simulink model "System"  (R2024a)
settings: Solver=VariableStepAuto  StartTime=0.0  StopTime=10.0  RelTol=1e-3
libraries: neural x2
settings Model: Creator=max11mus  LastModifiedBy=max11mus

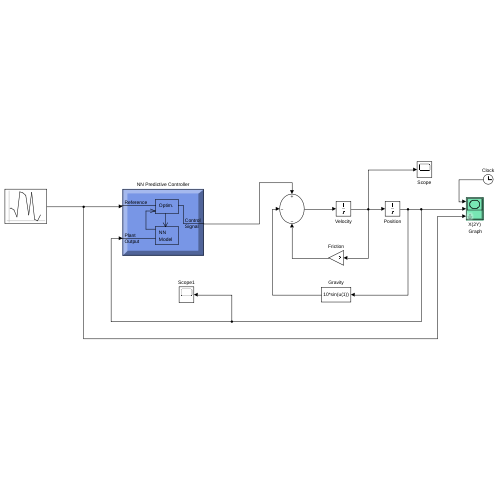
[thumbnail: Simulink's stored preview of the top-level diagram]
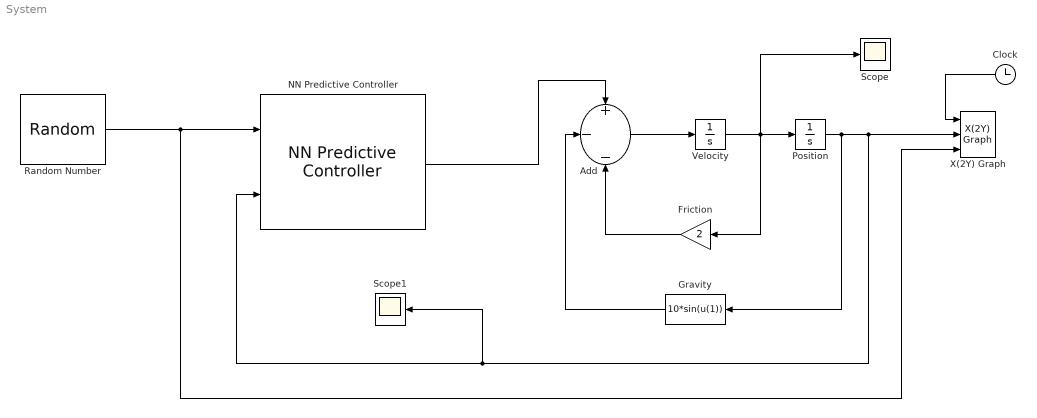
== system System ==
  Add : Sum  Inputs=+||-||-
  Clock : Clock
  Friction : Gain  Gain=2
  Gravity : Fcn  Expr=10*sin(u(1))
  NN Predictive Controller : neural/Control Systems/NN Predictive Controller  epochs=10  minp=-14.860973275977976016  maxp=14.972411842840820384  mint=-3.2887980026526069111  maxt=14.972411842840820384  Normalize=0  IW=[-0.032209844966698181201 0.0004842303811762906085 -0.038214774508017898547 0.087891959742595143767 -0.0049186837795332106343;-0.0037266038644475137781 -0.0053214205196589073679 0.006700009668674138455 0.0050755072350715437629 -0.0090455928933601964514;-0.0072756233672057243206 0.020376661347633842625 -0.033005692527208564668 0.010347523880553283898 0.036857966345246385986;-0.00038199302969159549571 -0.0059612728941718946124 0.013388867166121689797 -0.010360796205912608386 0.003487135037739601956;-0.0046614812815905194363 -0.0028269766095801204635 0.00030057352605401246783 0.0064554017982060268172 -0.0022030445024334051329;-0.0094467253000392586298 -0.0042207140094451646786 0.045248285726168152587 -0.025888487260812172164 -0.002820999804125486933;0.065543385541593959798 -0.0016025414154424494004 -0.0084955300195080837855 0.044609410010118671908 -0.26853262779806130744;0.017946126289430236467 -0.015971807856565621575 -0.0070211617130560765795 0.011444625729904966266 0.010874294340424636024;-0.0021688861781463536493 -0.0035622984387113317863 0.040072202786979448097 -0.018852965401898433978 -0.012267489590222301066;-0.0025428786120997304288 -0.0071555839750277652062 0.0052904364999521507826 0.004310034030136751515 -0.0029703349926871033468;0.007186386802497442966 0.0041023569100574761373 0.00068661195843568991956 -0.016977898377474390235 0.011745413647987718725;0.1130291466453810928 0.1847423194375882316 0.023123739836479410836 -0.2623344344032326747 -0.018356815139350751709;0.027774236790948012704 0.0028672682886705753644 0.015458774845652670932 -0.062765193394395860094 0.0054360877460552028961;0.0067224951938523978823 0.00083501283958491764187 -0.001283833296912832711 -0.012041984208070262777 0.0029837734768752635639;0.0069680791525584253807 -0.0044436167500601416597 0.0051584966512181230913 -0.014238832458994900992 -0.0051929494639878339204]  LW1_2=[-0.26243930864913889156 -0.12520756836498139752 -0.049859422322473881395 -0.0032752693913916230278 -0.21877664073705208048;-0.085553520951359610103 0.27651015843062082267 0.33749027304918660652 0.11372350823367174955 -0.13998821343616371649;-0.051262059060211306871 0.14553524371126419501 0.012158167251771118816 0.13234730689237414469 -0.31692057220921582283;-0.1659611043529373442 -0.22867683011507383695 -0.12064160820941764729 -0.25555605197606945378 0.47379167540947147996;-0.16667829573614167948 -0.14623179297968696977 -0.17550654818669228496 0.086019591308161766352 0.17447895641370442243;0.13273667574946193537 0.27597615594842184183 -0.12052646882881125345 0.15989614547386321597 -0.190668955400320278;0.013209872517279412987 0.17507718552719539473 -0.24607151945859806474 -0.084451465827836177946 -0.038421568456381463563;0.056189912372349971881 -0.19741810753112501442 0.015606879920724505903 0.023964644441251702067 0.24055696827493480705;0.25649967909796261845 0.053178233680966843777 0.18535281867337646822 -0.15204179248997790053 -0.10986325716373966654;-0.33505348193771761212 -0.19627538603327043809 0.130437673814499 -0.0097946347635215723348 0.12477419649646211142;0.14084781289795461623 -0.28347782651436276291 -0.28700933543676010462 0.1780649036607043767 -0.085136284393081823607;-0.2000008205941552486 -0.140154005050131647 0.027358468624533813923 0.072417932615793628726 -0.18151652074197416331;-0.26712085242982885891 0.17012835486666119666 0.16455985338081091651 0.20377306294523389596 -0.031959636277844219454;-0.28621748767442251049 -0.33565539170103531053 0.10951369435619884296 -0.28397325867506717501 0.36987661197218385523;-0.34568323062985784055 0.19495674497156445515 -0.33771385385234831134 -0.17879254297502281124 0.18187340190716883015]  LW2_1=[-0.19670780747207736172 0.48943971219372583992 0.05861849094253196446 -0.748363110144790733 -1.3207081283773423053 0.4996403819429138804 -0.0009330897574736068522 0.3050841234311010286 -0.10423990656781022268 -1.0592334664768505714 -0.38764689200030338911 -0.001259625694505661208 -0.24032878708955887626 -0.80806396659742874 -0.47954111583895159265]  B1=[1.6425792250629323021;1.4482182096917017855;1.1351168784748817409;-0.35189011592683427931;-1.0212524098312212306;0.22823606321288592014;0.25643926257357724241;-0.071686090700962171174;0.33622467913137360496;0.65380455810276194573;0.66630151988757357895;0.92733635674486480927;-1.4228939779206921656;1.4264035509661749934;-1.6916580195172119527]  B2=-0.73728098382225748519  max_i_int=2  min_i_int=0.1  limit_output=1  max_output=3.1  min_output=-3.1  Use_Previous_Weights=1  N2=[]  Nu=[]  Ts=0.05  rho=[]  alpha=[]  csrchfun=csrchbac  maxiter=[]  S1=15  Ni=5  Nj=5  sim_file=robotarm  trainfun=trainlm  Use_validation=1  Use_Testing=1  max_i=15  min_i=-15  sam_training=10000
  Position : Integrator
  Random Number : RandomNumber  SampleTime=0.1
  Scope : Scope
  Scope1 : Scope
  Velocity : Integrator
  X(2Y) Graph : neural/Control Systems/X(2Y)  Graph  xmin=0  xmax=5  ymin=21  ymax=22  st=-1
  wires:
  NN Predictive Controller/1 -> Add/1
  Add/1 -> Velocity/1
  Velocity/1 -> Scope/1, Friction/1, Position/1
  Position/1 -> Scope1/1, NN Predictive Controller/2, X(2Y) Graph/2, Gravity/1
  Friction/1 -> Add/3
  Gravity/1 -> Add/2
  Random Number/1 -> X(2Y) Graph/3, NN Predictive Controller/1
  Clock/1 -> X(2Y) Graph/1
